simulink model "EvPowertrainController4EM"  (R2023a)
settings: configuration reference "VehicleFixed10ms" (kept outside this file)
model workspace (MAT data in the model file):
  CtrlVcuCnstrntPnltyFctr = 10000000
  CtrlVcuEMTrqSplitGrid = 200
  CtrlVcuPwrDeltaPnlty = 2
  CtrlVcuTracPwrErrPnlty = 6
  CtrlVcuTrqVecBrkThresh = 0.01
  CtrlVcuTrqVecIGain = 0
  CtrlVcuTrqVecMinTrq = 50
  CtrlVcuTrqVecPGain = -2000
  CtrlVcuTrqVecSteerThresh = 0.349065850399
  CtrlVcuTrqVecVelThresh = 2.5
undefined symbols (not defined in the file): CtrlVcuEvChrgLmtBpt, CtrlVcuEvRegenBrkCutOff, CtrlVcuEvRegenBrkSpdBpt, CtrlVcuEvSocBpt, eff, PlntBrkActrBoreFrnt, PlntBrkFrntBias, PlntBrkKinFricCffFrnt, PlntBrkNumPadsFrnt, PlntBrkPadMeanRadiusFrnt, PlntBrkPrsFctr, PlntBrkRearBias, PlntDiffrntl2Eff, PlntDiffrntl2Ratio, PlntDiffrntlEff, PlntDiffrntlRatio, PlntEM1EffTbl, PlntEM1Spd, PlntEM1Trq, PlntEM1TrqEff, PlntEM2EffTbl, PlntEM2Spd, PlntEM2Trq, PlntEM2TrqEff, PlntEM3EffTbl, PlntEM3Spd, PlntEM3Trq, PlntEM3TrqEff, PlntEMWhlGearEffFL, PlntEMWhlGearEffRL, PlntEMWhlGearRatioFL, PlntEMWhlGearRatioRL, PlntTransEffSpdBpt, PlntTransEffTbl, PlntTransEffTempBpt, PlntTransEffTrqBpt, PlntTransGearNumVect, PlntTransGearRatioVect, PlntVehDstCGFrntAxl, PlntVehDstCGRearAxl, PlntWhlLdRadius
libraries: simulink x13, autolibutils x2, slpidlib x2
(part 1 of 5)
settings Model: DataDictionary=VirtualVehicleTemplate.sldd  ModifiedByFormat=The MathWorks, Inc.  Creator=The MathWorks, Inc.  LastModifiedBy=The MathWorks, Inc.
settings ConfigSetRef: SourceName=VehicleFixed10ms

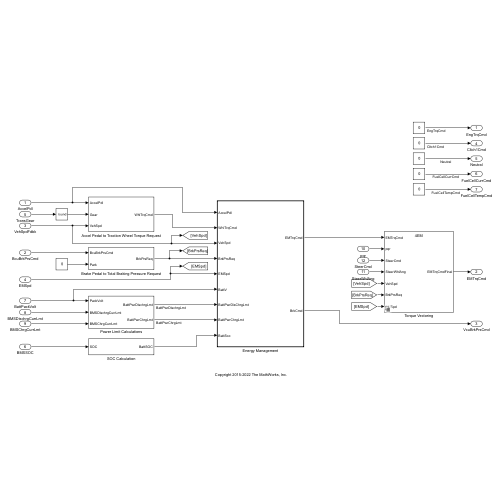
[thumbnail: Simulink's stored preview of the top-level diagram]
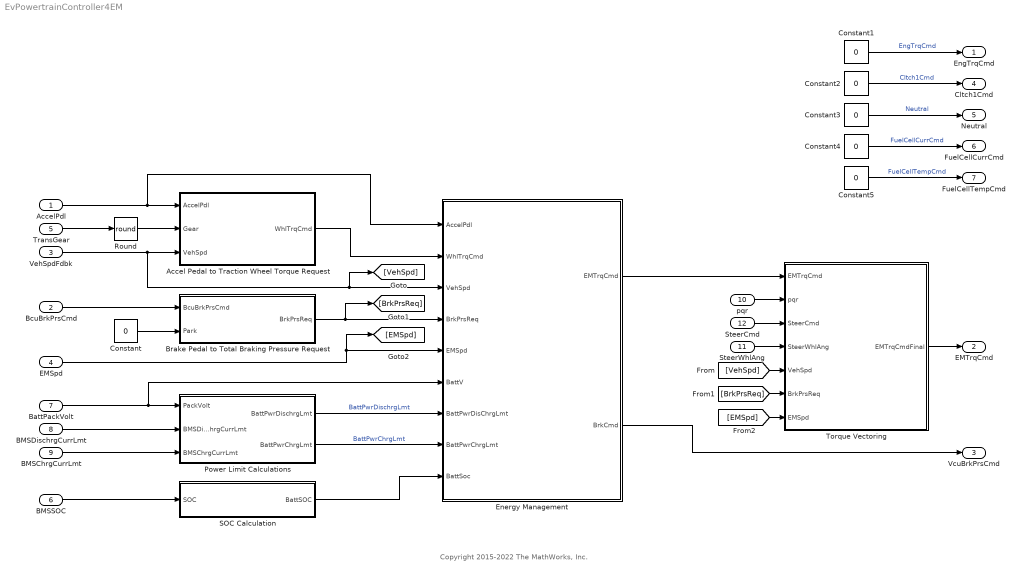
== system EvPowertrainController4EM ==
  note: Copyright 2015-2022 The MathWorks, Inc.
  AccelPdl : Inport  OutDataTypeStr=double  PortDimensions=1
  BcuBrkPrsCmd : Inport  Port=2  OutDataTypeStr=double  PortDimensions=4
  VehSpdFdbk : Inport  Port=3  OutDataTypeStr=double  PortDimensions=1
  EMSpd : Inport  Port=4  OutDataTypeStr=double
  TransGear : Inport  Port=5  OutDataTypeStr=double  PortDimensions=1
  BMSSOC : Inport  Port=6
  BattPackVolt : Inport  Port=7
  BMSDischrgCurrLmt : Inport  Port=8
  BMSChrgCurrLmt : Inport  Port=9
  pqr : Inport  Port=10  PortDimensions=3
  SteerWhlAng : Inport  Port=11  PortDimensions=4
  SteerCmd : Inport  Port=12
  Accel Pedal to Traction Wheel Torque Request : Subsystem  InitFcn=[~]=autosharedicon('autolibinternalvvblock',gcb,0);  VariantControl=Choice
  Brake Pedal to Total Braking Pressure Request : Subsystem  InitFcn=[~]=autosharedicon('autolibinternalvvblock',gcb,0);
  Constant : Constant  Value=0
  Constant{1..5} (5 alike) : Constant  Value=0  SampleTime=-1
  Energy Management : Subsystem  LoadFcn=[~]=autosharedicon('autolibinternalvvblock',gcb,0);  TreatAsAtomicUnit=on
  Power Limit Calculations : Subsystem  InitFcn=[~]=autosharedicon('autolibinternalvvblock',gcb,0);
  Round : Rounding  Operator=round
  SOC Calculation : Subsystem  InitFcn=[~]=autosharedicon('autolibinternalvvblock',gcb,0);
  Torque Vectoring : Subsystem  Variant=on  VariantControlMode=label  VariantControl=Choice  LabelModeActiveChoice=4EM
  EngTrqCmd : Outport  OutDataTypeStr=double  PortDimensions=1  VectorParamsAs1DForOutWhenUnconnected=off
  EMTrqCmd : Outport  Port=2  OutDataTypeStr=double  VectorParamsAs1DForOutWhenUnconnected=off
  VcuBrkPrsCmd : Outport  Port=3  OutDataTypeStr=double  PortDimensions=4  VectorParamsAs1DForOutWhenUnconnected=off
  Cltch1Cmd : Outport  Port=4  OutDataTypeStr=double  PortDimensions=1  VectorParamsAs1DForOutWhenUnconnected=off
  Neutral : Outport  Port=5  OutDataTypeStr=double  PortDimensions=1  VectorParamsAs1DForOutWhenUnconnected=off
  FuelCellCurrCmd : Outport  Port=6  OutDataTypeStr=double  PortDimensions=1
  FuelCellTempCmd : Outport  Port=7  OutDataTypeStr=double  PortDimensions=1
  wires:
  AccelPdl/1 -> Energy Management/1(AccelPdl), Accel Pedal to Traction Wheel Torque Request/1(AccelPdl)
  BcuBrkPrsCmd/1 -> Brake Pedal to Total Braking Pressure Request/1(BcuBrkPrsCmd)
  Energy Management/2(BrkCmd) -> VcuBrkPrsCmd/1
  Constant/1 -> Brake Pedal to Total Braking Pressure Request/2(Park)
  Brake Pedal to Total Braking Pressure Request/1(BrkPrsReq) -> [BrkPrsReq], Energy Management/4("BrkPrsReq ")
  VehSpdFdbk/1 -> [VehSpd], Energy Management/3(VehSpd), Accel Pedal to Traction Wheel Torque Request/3(VehSpd)
  Constant2/1 -> Cltch1Cmd/1  "Cltch1Cmd"
  Constant3/1 -> Neutral/1  "Neutral"
  Constant1/1 -> EngTrqCmd/1  "EngTrqCmd"
  Constant4/1 -> FuelCellCurrCmd/1  "FuelCellCurrCmd"
  Constant5/1 -> FuelCellTempCmd/1  "FuelCellTempCmd"
  Accel Pedal to Traction Wheel Torque Request/1(WhlTrqCmd) -> Energy Management/2(WhlTrqCmd)
  TransGear/1 -> Round/1
  Round/1 -> Accel Pedal to Traction Wheel Torque Request/2(Gear)
  BMSChrgCurrLmt/1 -> Power Limit Calculations/3(BMSChrgCurrLmt)
  BMSSOC/1 -> SOC Calculation/1(SOC)
  BattPackVolt/1 -> Energy Management/6(BattV), Power Limit Calculations/1(PackVolt)
  BMSDischrgCurrLmt/1 -> Power Limit Calculations/2(BMSDischrgCurrLmt)
  Power Limit Calculations/1(BattPwrDischrgLmt) -> Energy Management/7(BattPwrDisChrgLmt)  "BattPwrDischrgLmt"
  Power Limit Calculations/2(BattPwrChrgLmt) -> Energy Management/8("BattPwrChrgLmt ")  "BattPwrChrgLmt"
  SOC Calculation/1(BattSOC) -> Energy Management/9(BattSoc)
  EMSpd/1 -> [EMSpd], Energy Management/5(EMSpd)
  Energy Management/1(EMTrqCmd) -> Torque Vectoring/1(EMTrqCmd)
  pqr/1 -> Torque Vectoring/2(pqr)
  SteerCmd/1 -> Torque Vectoring/3(SteerCmd)
  SteerWhlAng/1 -> Torque Vectoring/4(SteerWhlAng)
  [VehSpd] -> Torque Vectoring/5(VehSpd)
  [BrkPrsReq] -> Torque Vectoring/6(BrkPrsReq)
  [EMSpd] -> Torque Vectoring/7(EMSpd)
  Torque Vectoring/1(EMTrqCmdFinal) -> EMTrqCmd/1

== system EvPowertrainController4EM/Accel Pedal to Traction Wheel Torque Request ==
  note: Convert Accelerator Pedal Position to
      | Wheel Torque Command using Motor
      | Torque Speed Curves.
      |
      | Can be replaced with 2D Lookup Table
      | with AccelPdl and VehSpd as inputs and
      | Motor or Wheel Torque Command as output.
  AccelPdl : Inport
  Gear : Inport  Port=2
  VehSpd : Inport  Port=3
  EM2WhlTrq : Subsystem  Variant=on  VariantControlMode=label  VariantControl=Choice  LabelModeActiveChoice=4EM
  Product1 : Product
  WhlTrqCmd : Outport  VectorParamsAs1DForOutWhenUnconnected=off
  wires:
  Product1/1 -> WhlTrqCmd/1
  AccelPdl/1 -> Product1/1
  Gear/1 -> EM2WhlTrq/1(Gear)
  VehSpd/1 -> EM2WhlTrq/2(VehSpd)
  EM2WhlTrq/1(WhlTrqCmd) -> Product1/2

== system EvPowertrainController4EM/Brake Pedal to Total Braking Pressure Request ==
  BcuBrkPrsCmd : Inport
  Park : Inport  Port=2
  Front Bias : Constant  Value=PlntBrkFrntBias
  Gain4 : Gain  Gain=PlntBrkPrsFctr
  Mux : Mux
  Product : Product
  Rear Bias : Constant  Value=PlntBrkRearBias
  Terminator : Terminator
  BrkPrsReq : Outport  VectorParamsAs1DForOutWhenUnconnected=off
  wires:
  BcuBrkPrsCmd/1 -> Product/2
  Mux/1 -> Product/1
  Rear Bias/1 -> Mux/4, Mux/3
  Front Bias/1 -> Mux/1, Mux/2
  Gain4/1 -> BrkPrsReq/1
  Product/1 -> Gain4/1
  Park/1 -> Terminator/1

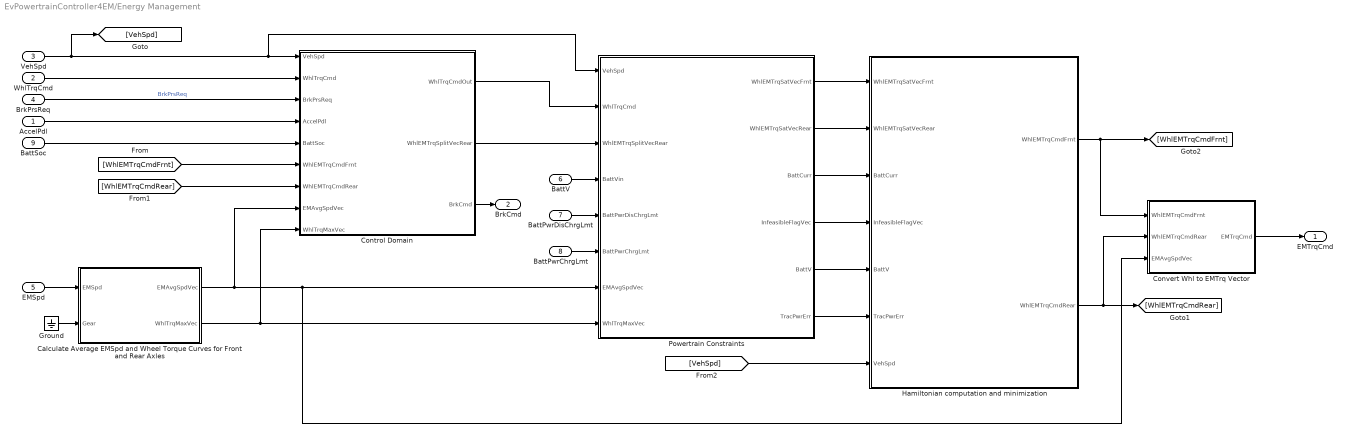
== system EvPowertrainController4EM/Energy Management ==
  AccelPdl : Inport
  WhlTrqCmd : Inport  Port=2
  VehSpd : Inport  Port=3
  "BrkPrsReq " : Inport  Port=4
  EMSpd : Inport  Port=5
  BattV : Inport  Port=6
  BattPwrDisChrgLmt : Inport  Port=7
  "BattPwrChrgLmt " : Inport  Port=8
  BattSoc : Inport  Port=9
  Calculate Average EMSpd and Wheel Torque Curves for Front and Rear Axles : Subsystem  Variant=on  VariantControlMode=label  VariantControl=Choice  LabelModeActiveChoice=4EM
  "Control Domain " : Subsystem  InitFcn="[~] =  autosharedeval('1');"
  Convert Whl to EMTrq Vector : Subsystem  Variant=on  VariantControlMode=label  VariantControl=Choice  LabelModeActiveChoice=4EM
  Ground : Ground
  Hamiltonian computation and minimization : Subsystem  InitFcn="[~] =  autosharedeval('1');"
  "Powertrain Constraints " : Subsystem  InitFcn="[~] =  autosharedeval('1');"
  EMTrqCmd : Outport  VectorParamsAs1DForOutWhenUnconnected=off
  BrkCmd : Outport  Port=2  VectorParamsAs1DForOutWhenUnconnected=off
  wires:
  "Control Domain "/1(WhlTrqCmdOut) -> "Powertrain Constraints "/2(WhlTrqCmd)
  "BrkPrsReq "/1 -> "Control Domain "/3("BrkPrsReq ")  "BrkPrsReq"
  AccelPdl/1 -> "Control Domain "/4(AccelPdl)
  "Control Domain "/3(BrkCmd) -> BrkCmd/1
  "Powertrain Constraints "/6(TracPwrErr) -> Hamiltonian computation and minimization/6(TracPwrErr)
  BattV/1 -> "Powertrain Constraints "/4(BattVin)
  VehSpd/1 -> [VehSpd], "Control Domain "/1(VehSpd), "Powertrain Constraints "/1(VehSpd)
  Hamiltonian computation and minimization/2(WhlEMTrqCmdRear) -> [WhlEMTrqCmdRear], Convert Whl to EMTrq Vector/2(WhlEMTrqCmdRear)
  Hamiltonian computation and minimization/1(WhlEMTrqCmdFrnt) -> [WhlEMTrqCmdFrnt], Convert Whl to EMTrq Vector/1(WhlEMTrqCmdFrnt)
  "Powertrain Constraints "/4(InfeasibleFlagVec) -> Hamiltonian computation and minimization/4(InfeasibleFlagVec)
  "Powertrain Constraints "/3(BattCurr) -> Hamiltonian computation and minimization/3(BattCurr)
  "Powertrain Constraints "/5(BattV) -> Hamiltonian computation and minimization/5(BattV)
  WhlTrqCmd/1 -> "Control Domain "/2(WhlTrqCmd)
  "Control Domain "/2(WhlEMTrqSplitVecRear) -> "Powertrain Constraints "/3(WhlEMTrqSplitVecRear)
  Calculate Average EMSpd and Wheel Torque Curves for Front and Rear Axles/1(EMAvgSpdVec) -> Convert Whl to EMTrq Vector/3(EMAvgSpdVec), "Powertrain Constraints "/7(EMAvgSpdVec), "Control Domain "/8(EMAvgSpdVec)
  "BattPwrChrgLmt "/1 -> "Powertrain Constraints "/6("BattPwrChrgLmt ")
  BattPwrDisChrgLmt/1 -> "Powertrain Constraints "/5(BattPwrDisChrgLmt)
  [WhlEMTrqCmdFrnt] -> "Control Domain "/6(WhlEMTrqCmdFrnt)
  BattSoc/1 -> "Control Domain "/5(BattSoc)
  EMSpd/1 -> Calculate Average EMSpd and Wheel Torque Curves for Front and Rear Axles/1(EMSpd)
  Convert Whl to EMTrq Vector/1(EMTrqCmd) -> EMTrqCmd/1
  [WhlEMTrqCmdRear] -> "Control Domain "/7(WhlEMTrqCmdRear)
  Ground/1 -> Calculate Average EMSpd and Wheel Torque Curves for Front and Rear Axles/2(Gear)
  Calculate Average EMSpd and Wheel Torque Curves for Front and Rear Axles/2(WhlTrqMaxVec) -> "Powertrain Constraints "/8(WhlTrqMaxVec), "Control Domain "/9(WhlTrqMaxVec)
  "Powertrain Constraints "/1(WhlEMTrqSatVecFrnt) -> Hamiltonian computation and minimization/1(WhlEMTrqSatVecFrnt)
  "Powertrain Constraints "/2(WhlEMTrqSatVecRear) -> Hamiltonian computation and minimization/2(WhlEMTrqSatVecRear)
  [VehSpd] -> Hamiltonian computation and minimization/7(VehSpd)

== system EvPowertrainController4EM/Power Limit Calculations ==
  note: BMS has opposite sign convention for current
  note: Use Current Limits from BMS to calculate
      | discharge and charge power limits
  PackVolt : Inport
  BMSDischrgCurrLmt : Inport  Port=2
  BMSChrgCurrLmt : Inport  Port=3
  Data Type Conversion : DataTypeConversion  SaturateOnIntegerOverflow=off  RndMeth=Floor
  Data Type Conversion1 : DataTypeConversion  SaturateOnIntegerOverflow=off  RndMeth=Floor
  Gain : Gain  Gain=-1
  Gain1 : Gain  Gain=-1
  Product : Product
  Product1 : Product
  BattPwrDischrgLmt : Outport  VectorParamsAs1DForOutWhenUnconnected=off
  BattPwrChrgLmt : Outport  Port=2  VectorParamsAs1DForOutWhenUnconnected=off
  wires:
  Gain/1 -> Product1/2
  Gain1/1 -> Product/2
  Product/1 -> Data Type Conversion1/1
  Product1/1 -> Data Type Conversion/1
  PackVolt/1 -> Product/1, Product1/1
  BMSChrgCurrLmt/1 -> Gain/1
  BMSDischrgCurrLmt/1 -> Gain1/1
  Data Type Conversion/1 -> BattPwrChrgLmt/1
  Data Type Conversion1/1 -> BattPwrDischrgLmt/1

== system EvPowertrainController4EM/SOC Calculation ==
  SOC : Inport
  Data Type Conversion : DataTypeConversion  SaturateOnIntegerOverflow=off  RndMeth=Floor
  convert2percent : Gain  Gain=100
  BattSOC : Outport
  wires:
  convert2percent/1 -> Data Type Conversion/1
  SOC/1 -> convert2percent/1
  Data Type Conversion/1 -> BattSOC/1

== system EvPowertrainController4EM/Torque Vectoring ==
  EMTrqCmd : Inport
  pqr : Inport  Port=2
  SteerCmd : Inport  Port=3
  SteerWhlAng : Inport  Port=4
  VehSpd : Inport  Port=5
  BrkPrsReq : Inport  Port=6
  EMSpd : Inport  Port=7
  3EM : Subsystem  LoadFcn=[~]=autosharedicon('autolibinternalvvblock',gcb,0);  VariantControl=3EM
  4EM : Subsystem  LoadFcn=[~]=autosharedicon('autolibinternalvvblock',gcb,0);  VariantControl=4EM
  No Torque Vectoring : Subsystem  VariantControl=No Torque Vectoring
  EMTrqCmdFinal : Outport

== system EvPowertrainController4EM/Accel Pedal to Traction Wheel Torque Request/EM2WhlTrq ==
  Gear : Inport
  VehSpd : Inport  Port=2
  2EM : Subsystem  VariantControl=2EM
  3EM Dual Front : Subsystem  VariantControl=3EM Dual Front
  3EM Dual Rear : Subsystem  VariantControl=3EM Dual Rear
  4EM : Subsystem  VariantControl=4EM
  WhlTrqCmd : Outport

== system EvPowertrainController4EM/Energy Management/Calculate Average EMSpd and Wheel Torque Curves for Front and Rear Axles ==
  EMSpd : Inport
  Gear : Inport  Port=2
  2EM : Subsystem  VariantControl=2EM
  3EM Dual Front : Subsystem  VariantControl=3EM Dual Front
  3EM Dual Rear : Subsystem  VariantControl=3EM Dual Rear
  4EM : Subsystem  VariantControl=4EM
  EMAvgSpdVec : Outport
  WhlTrqMaxVec : Outport  Port=2

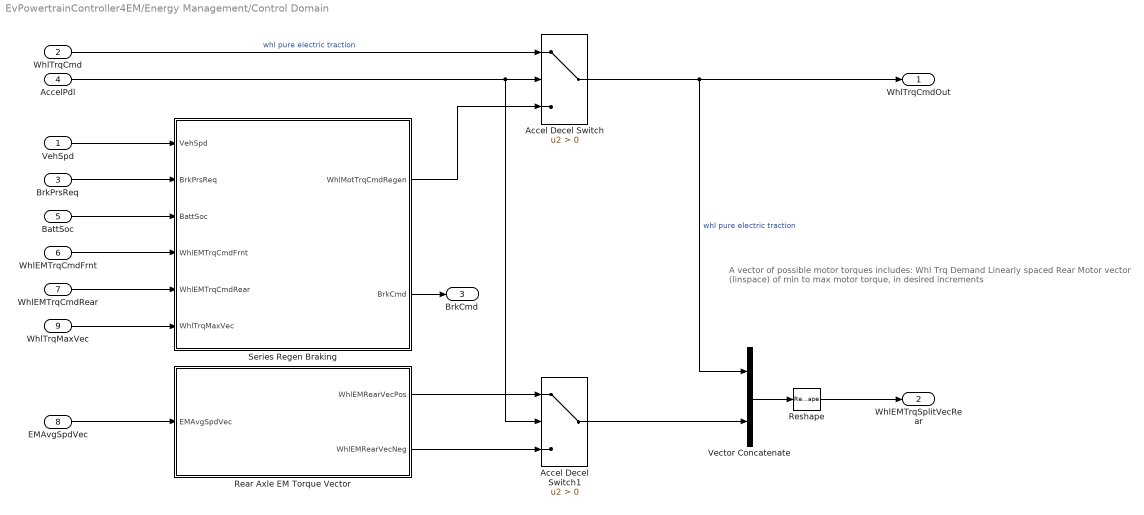
== system EvPowertrainController4EM/Energy Management/Control Domain  ==
  note: A vector of possible motor torques includes:
      | Whl Trq Demand
      | Linearly spaced Rear Motor vector (linspace) of min to max motor torque, in desired increments
  VehSpd : Inport
  WhlTrqCmd : Inport  Port=2
  "BrkPrsReq " : Inport  Port=3
  AccelPdl : Inport  Port=4
  BattSoc : Inport  Port=5
  WhlEMTrqCmdFrnt : Inport  Port=6
  WhlEMTrqCmdRear : Inport  Port=7
  EMAvgSpdVec : Inport  Port=8
  WhlTrqMaxVec : Inport  Port=9
  Accel Decel Switch : Switch  Criteria=u2 > Threshold  SaturateOnIntegerOverflow=off  InputSameDT=off
  Accel Decel Switch1 : Switch  Criteria=u2 > Threshold  SaturateOnIntegerOverflow=off  InputSameDT=off
  Rear Axle EM Torque Vector : Subsystem  Variant=on  VariantControlMode=label  VariantControl=Choice  LabelModeActiveChoice=3EM Dual Rear or 4EM
  Reshape : Reshape
  Series Regen Braking : Subsystem  InitFcn=%[~]=autosharedicon('autolibutils',gcb,0);  VariantControl=Variant
  Vector Concatenate : Concatenate
  WhlTrqCmdOut : Outport  VectorParamsAs1DForOutWhenUnconnected=off
  WhlEMTrqSplitVecRear : Outport  Port=2  VectorParamsAs1DForOutWhenUnconnected=off
  BrkCmd : Outport  Port=3  VectorParamsAs1DForOutWhenUnconnected=off
  wires:
  Vector Concatenate/1 -> Reshape/1
  Reshape/1 -> WhlEMTrqSplitVecRear/1
  WhlTrqMaxVec/1 -> Series Regen Braking/6(WhlTrqMaxVec)
  AccelPdl/1 -> Accel Decel Switch1/2, Accel Decel Switch/2
  Series Regen Braking/2(" BrkCmd") -> BrkCmd/1
  WhlTrqCmd/1 -> Accel Decel Switch/1  "whl pure electric traction"
  "BrkPrsReq "/1 -> Series Regen Braking/2("BrkPrsReq ")
  EMAvgSpdVec/1 -> Rear Axle EM Torque Vector/1(EMAvgSpdVec)
  VehSpd/1 -> Series Regen Braking/1(VehSpd)
  Accel Decel Switch/1 -> Vector Concatenate/1, WhlTrqCmdOut/1  "whl pure electric traction"
  Accel Decel Switch1/1 -> Vector Concatenate/2
  Series Regen Braking/1(" WhlMotTrqCmdRegen") -> Accel Decel Switch/3
  WhlEMTrqCmdFrnt/1 -> Series Regen Braking/4(WhlEMTrqCmdFrnt)
  WhlEMTrqCmdRear/1 -> Series Regen Braking/5(WhlEMTrqCmdRear)
  BattSoc/1 -> Series Regen Braking/3(BattSoc)
  Rear Axle EM Torque Vector/1(WhlEMRearVecPos) -> Accel Decel Switch1/1
  Rear Axle EM Torque Vector/2(WhlEMRearVecNeg) -> Accel Decel Switch1/3

== system EvPowertrainController4EM/Energy Management/Convert Whl to EMTrq Vector ==
  WhlEMTrqCmdFrnt : Inport
  WhlEMTrqCmdRear : Inport  Port=2
  EMAvgSpdVec : Inport  Port=3
  2EM : Subsystem  VariantControl=2EM
  3EM Dual Front : Subsystem  VariantControl=3EM Dual Front
  3EM Dual Rear : Subsystem  VariantControl=3EM Dual Rear
  4EM : Subsystem  VariantControl=4EM
  EMTrqCmd : Outport

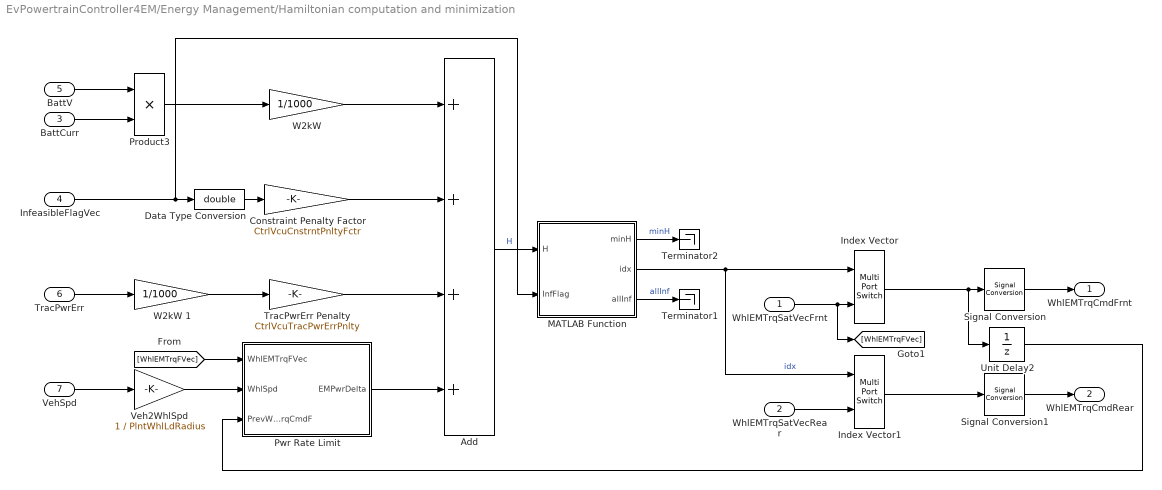
== system EvPowertrainController4EM/Energy Management/Hamiltonian computation and minimization ==
  WhlEMTrqSatVecFrnt : Inport
  WhlEMTrqSatVecRear : Inport  Port=2
  BattCurr : Inport  Port=3
  InfeasibleFlagVec : Inport  Port=4
  BattV : Inport  Port=5
  TracPwrErr : Inport  Port=6
  VehSpd : Inport  Port=7
  Add : Sum  Inputs=++++
  Constraint Penalty Factor : Gain  Gain=CtrlVcuCnstrntPnltyFctr
  Data Type Conversion : DataTypeConversion  OutDataTypeStr=double  SaturateOnIntegerOverflow=off  RndMeth=Floor
  Index Vector : MultiPortSwitch  Inputs=1  SaturateOnIntegerOverflow=off  InputSameDT=off
  Index Vector1 : MultiPortSwitch  Inputs=1  SaturateOnIntegerOverflow=off  InputSameDT=off
  MATLAB Function : MATLAB Function  InitFcn="[~] =  autosharedeval('1');"  TreatAsAtomicUnit=on
  Product3 : Product
  Pwr Rate Limit : Subsystem  InitFcn="[~] =  autosharedeval('1');"
  Signal Conversion : SignalConversion  OverrideOpt=off
  Signal Conversion1 : SignalConversion  OverrideOpt=off
  Terminator1 : Terminator
  Terminator2 : Terminator
  TracPwrErr Penalty : Gain  Gain=CtrlVcuTracPwrErrPnlty
  Unit Delay2 : UnitDelay  SampleTime=-1  HasFrameUpgradeWarning=on
  Veh2WhlSpd : Gain  Gain=1 / PlntWhlLdRadius
  "W2kW " : Gain  Gain=1/1000
  W2kW 1 : Gain  Gain=1/1000
  WhlEMTrqCmdFrnt : Outport  VectorParamsAs1DForOutWhenUnconnected=off
  WhlEMTrqCmdRear : Outport  Port=2  VectorParamsAs1DForOutWhenUnconnected=off
  wires:
  Constraint Penalty Factor/1 -> Add/2
  TracPwrErr Penalty/1 -> Add/3
  W2kW 1/1 -> TracPwrErr Penalty/1
  TracPwrErr/1 -> W2kW 1/1
  Signal Conversion1/1 -> WhlEMTrqCmdRear/1
  Signal Conversion/1 -> WhlEMTrqCmdFrnt/1
  Index Vector/1 -> Unit Delay2/1, Signal Conversion/1
  "W2kW "/1 -> Add/1
  BattV/1 -> Product3/1
  BattCurr/1 -> Product3/2
  Index Vector1/1 -> Signal Conversion1/1
  Add/1 -> MATLAB Function/1(H)  "H"
  MATLAB Function/1(minH) -> Terminator2/1  "minH"
  MATLAB Function/2(idx) -> Index Vector1/1, Index Vector/1  "idx"
  WhlEMTrqSatVecRear/1 -> Index Vector1/2
  InfeasibleFlagVec/1 -> Data Type Conversion/1, MATLAB Function/2(InfFlag)
  WhlEMTrqSatVecFrnt/1 -> Index Vector/2, [WhlEMTrqFVec]
  Product3/1 -> "W2kW "/1
  [WhlEMTrqFVec] -> Pwr Rate Limit/1(WhlEMTrqFVec)
  Veh2WhlSpd/1 -> Pwr Rate Limit/2(WhlSpd)
  Unit Delay2/1 -> Pwr Rate Limit/3(PrevWhlEMTrqCmdF)
  MATLAB Function/3(allInf) -> Terminator1/1  "allInf"
  Pwr Rate Limit/1(EMPwrDelta) -> Add/4
  Data Type Conversion/1 -> Constraint Penalty Factor/1
  VehSpd/1 -> Veh2WhlSpd/1

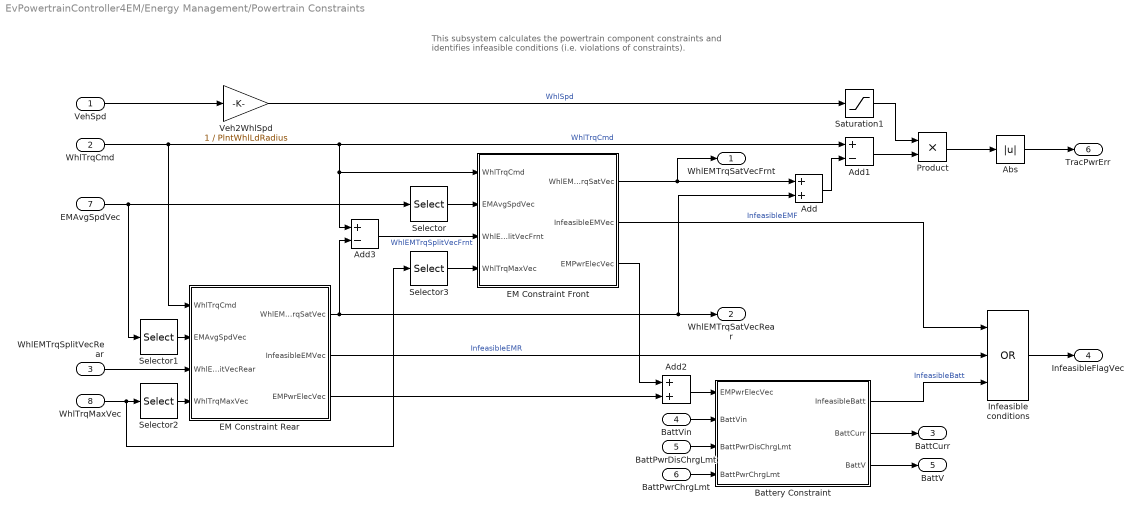
== system EvPowertrainController4EM/Energy Management/Powertrain Constraints  ==
  note: This subsystem calculates the powertrain component constraints
      | and identifies infeasible conditions (i.e. violations of constraints).
  VehSpd : Inport
  WhlTrqCmd : Inport  Port=2
  WhlEMTrqSplitVecRear : Inport  Port=3
  BattVin : Inport  Port=4
  BattPwrDisChrgLmt : Inport  Port=5
  "BattPwrChrgLmt " : Inport  Port=6
  EMAvgSpdVec : Inport  Port=7
  WhlTrqMaxVec : Inport  Port=8
  Abs : Abs  SaturateOnIntegerOverflow=off
  Add : Sum
  Add1 : Sum  Inputs=+-
  Add2 : Sum
  Add3 : Sum  Inputs=+-
  Battery Constraint : Subsystem  InitFcn="[~] =  autosharedeval('1');"
  EM Constraint Front : Subsystem  InitFcn="[~] =  autosharedeval('1');"
  EM Constraint Rear : Subsystem  InitFcn="[~] =  autosharedeval('1');"
  Infeasible conditions : Logic  Operator=OR  Inputs=3  AllPortsSameDT=off  OutDataTypeStr=boolean
  Product : Product
  Saturation1 : Saturate  UpperLimit=inf  LowerLimit=0.001
  Selector : Selector  InputPortWidth=2  IndexOptions=Index vector (dialog)  Indices=[1]  OutputSizes=1
  Selector1 : Selector  InputPortWidth=2  IndexOptions=Index vector (dialog)  Indices=[2]  OutputSizes=1
  Selector2 : Selector  InputPortWidth=2  IndexOptions=Index vector (dialog)  Indices=[2]  OutputSizes=1
  Selector3 : Selector  InputPortWidth=2  IndexOptions=Index vector (dialog)  Indices=[1]  OutputSizes=1
  Veh2WhlSpd : Gain  Gain=1 / PlntWhlLdRadius
  WhlEMTrqSatVecFrnt : Outport  VectorParamsAs1DForOutWhenUnconnected=off
  WhlEMTrqSatVecRear : Outport  Port=2  VectorParamsAs1DForOutWhenUnconnected=off
  BattCurr : Outport  Port=3  VectorParamsAs1DForOutWhenUnconnected=off
  InfeasibleFlagVec : Outport  Port=4  VectorParamsAs1DForOutWhenUnconnected=off
  BattV : Outport  Port=5  VectorParamsAs1DForOutWhenUnconnected=off
  TracPwrErr : Outport  Port=6  VectorParamsAs1DForOutWhenUnconnected=off
  wires:
  EM Constraint Rear/1(WhlEMTrqSatVec) -> WhlEMTrqSatVecRear/1, Add/2, Add3/2
  Add/1 -> Add1/2
  Add1/1 -> Product/2
  Battery Constraint/1(InfeasibleBatt) -> Infeasible conditions/3  "InfeasibleBatt"
  Infeasible conditions/1 -> InfeasibleFlagVec/1
  EM Constraint Rear/2(InfeasibleEMVec) -> Infeasible conditions/2  "InfeasibleEMR"
  Abs/1 -> TracPwrErr/1
  Veh2WhlSpd/1 -> Saturation1/1  "WhlSpd"
  Saturation1/1 -> Product/1
  BattVin/1 -> Battery Constraint/2(BattVin)
  WhlTrqCmd/1 -> EM Constraint Rear/1(WhlTrqCmd), Add1/1, EM Constraint Front/1(WhlTrqCmd), Add3/1  "WhlTrqCmd"
  WhlEMTrqSplitVecRear/1 -> EM Constraint Rear/3(WhlEMTrqSplitVecRear)
  EM Constraint Front/1(WhlEMTrqSatVec) -> WhlEMTrqSatVecFrnt/1, Add/1
  Battery Constraint/2(BattCurr) -> BattCurr/1
  EM Constraint Front/2(InfeasibleEMVec) -> Infeasible conditions/1  "InfeasibleEMF"
  Add2/1 -> Battery Constraint/1(EMPwrElecVec)
  VehSpd/1 -> Veh2WhlSpd/1
  EM Constraint Rear/3(EMPwrElecVec) -> Add2/2
  Battery Constraint/3(BattV) -> BattV/1
  EMAvgSpdVec/1 -> Selector/1, Selector1/1
  Add3/1 -> EM Constraint Front/3(WhlEMTrqSplitVecFrnt)  "WhlEMTrqSplitVecFrnt"
  Product/1 -> Abs/1
  EM Constraint Front/3(EMPwrElecVec) -> Add2/1
  "BattPwrChrgLmt "/1 -> Battery Constraint/4("BattPwrChrgLmt ")
  BattPwrDisChrgLmt/1 -> Battery Constraint/3(BattPwrDisChrgLmt)
  WhlTrqMaxVec/1 -> Selector3/1, Selector2/1
  Selector/1 -> EM Constraint Front/2(EMAvgSpdVec)
  Selector1/1 -> EM Constraint Rear/2(EMAvgSpdVec)
  Selector2/1 -> EM Constraint Rear/4(WhlTrqMaxVec)
  Selector3/1 -> EM Constraint Front/4(WhlTrqMaxVec)

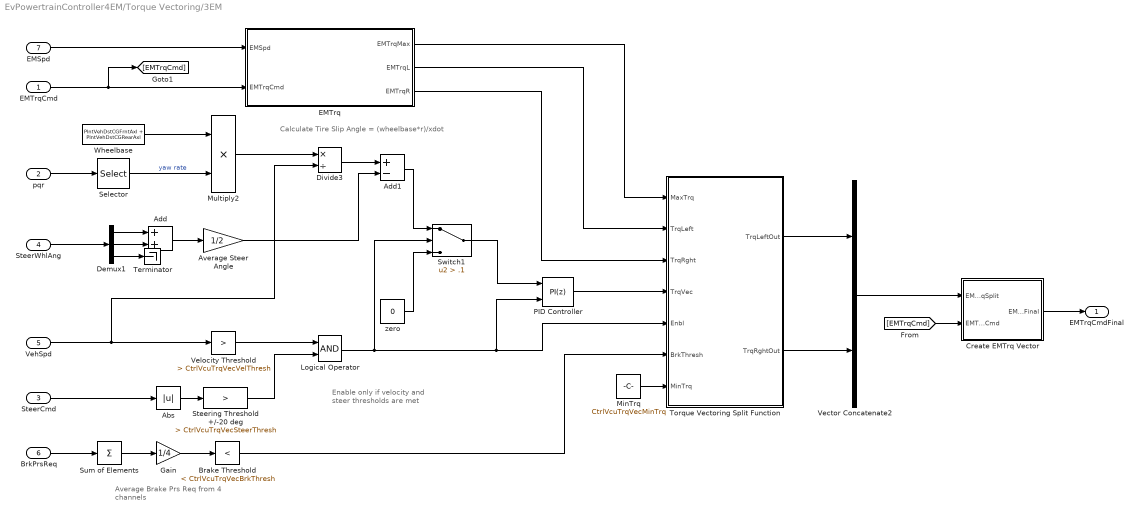
== system EvPowertrainController4EM/Torque Vectoring/3EM ==
  note: Calculate Tire Slip Angle = (wheelbase*r)/xdot
  note: Enable only if velocity and
      | steer thresholds are met
  note: Average Brake Prs Req
      | from 4 channels
  EMTrqCmd : Inport
  pqr : Inport  Port=2
  SteerCmd : Inport  Port=3
  SteerWhlAng : Inport  Port=4
  VehSpd : Inport  Port=5
  BrkPrsReq : Inport  Port=6
  EMSpd : Inport  Port=7
  Abs : Abs  SaturateOnIntegerOverflow=off
  Add : Sum
  Add1 : Sum  Inputs=+-
  Average Steer Angle : Gain  Gain=1/2
  Brake Threshold : simulink/Logic and Bit Operations/Compare To Constant  relop=<  const=CtrlVcuTrqVecBrkThresh  OutDataTypeStr=boolean
  Create EMTrq Vector : Subsystem  Variant=on  VariantControlMode=label  VariantControl=Choice  LabelModeActiveChoice=3EMDualRear
  Demux1 : Demux  Outputs=[1 1 2]
  Divide3 : Product  Inputs=*/
  EMTrq : Subsystem  Variant=on  VariantControlMode=label  VariantControl=Choice  LabelModeActiveChoice=3EMDualRear
  Gain : Gain  Gain=1/4
  Logical Operator : Logic  AllPortsSameDT=off  OutDataTypeStr=boolean
  MinTrq : Constant  Value=CtrlVcuTrqVecMinTrq  SampleTime=-1
  Multiply2 : Product
  PID Controller : slpidlib/PID Controller  Controller=PI  Form=Parallel  TimeDomain=Discrete-time  UseExternalTs=off  SampleTime=-1  IntegratorMethod=Forward Euler  FilterMethod=Forward Euler  ControllerParametersSource=internal  P=CtrlVcuTrqVecPGain  I=CtrlVcuTrqVecPGain  UseKiTs=off  D=0  N=1  UseFilter=on  TunerSelectOption=Transfer Function Based (PID Tuner App)  ZeroCross=off  InitialConditionSource=internal  InitialConditionForIntegrator=0  InitialConditionForFilter=0  DifferentiatorICPrevScaledInput=0  ExternalReset=either  TrackingMode=off  Kt=1  LimitOutput=off  SatLimitsSource=internal  UpperSaturationLimit=inf  LowerSaturationLimit=-inf  LinearizeAsGain=on  AntiWindupMode=none  Kb=1  LimitIntegrator=off  UpperIntegratorSaturationLimit=inf  LowerIntegratorSaturationLimit=-inf  POutMin=[]  POutMax=[]  IOutMin=[]  IOutMax=[]  DOutMin=[]  DOutMax=[]  NOutMin=[]  NOutMax=[]  SumOutMin=[]  SumOutMax=[]  SaturationOutMin=[]  SaturationOutMax=[]  PParamMin=[]  PParamMax=[]  IParamMin=[]  IParamMax=[]  DParamMin=[]  DParamMax=[]  NParamMin=[]  NParamMax=[]  KbParamMin=[]  KbParamMax=[]  KtParamMin=[]  KtParamMax=[]  KbOutMin=[]  KbOutMax=[]  KtOutMin=[]  KtOutMax=[]  IntegratorOutMin=[]  IntegratorOutMax=[]  FilterOutMin=[]  FilterOutMax=[]  SumI1OutMin=[]  SumI1OutMax=[]  SumI2OutMin=[]  SumI2OutMax=[]  SumI3OutMin=[]  SumI3OutMax=[]  SumI4OutMin=[]  SumI4OutMax=[]  SumDOutMin=[]  SumDOutMax=[]  DifferentiatorOutMin=[]  DifferentiatorOutMax=[]  FilterDiffOutCoefMin=[]  FilterDiffOutCoefMax=[]  ReciprocalOutMin=[]  ReciprocalOutMax=[]  SumDenOutMin=[]  SumDenOutMax=[]  SumNumOutMin=[]  SumNumOutMax=[]  DivideOutMin=[]  DivideOutMax=[]  UdiffTsProdOutMin=[]  UdiffTsProdOutMax=[]  NTsProdOutMin=[]  NTsProdOutMax=[]  UintegralTsProdOutMin=[]  UintegralTsProdOutMax=[]  UngainTsProdOutMin=[]  UngainTsProdOutMax=[]  ClampingZeroOutDataTypeStr=Inherit: Inherit via back propagation  ClampingZeroOutMin=[]  ClampingZeroOutMax=[]  FilterDenConstantOutDataTypeStr=Inherit: Inherit via back propagation  FilterDenConstantOutMin=[]  FilterDenConstantOutMax=[]  PCopyOutDataTypeStr=Inherit: Inherit via back propagation  PCopyOutMin=[]  PCopyOutMax=[]  NCopyOutDataTypeStr=Inherit: Inherit via back propagation  NCopyOutMin=[]  NCopyOutMax=[]  IntegratorContinuousStateAttributes=''  IntegratorStateMustResolveToSignalObject=off  IntegratorRTWStateStorageClass=Auto  FilterContinuousStateAttributes=''  FilterStateMustResolveToSignalObject=off  FilterRTWStateStorageClass=Auto  ParallelPVariant=InternalParameters  IdealPVariant=Disabled  IVariant=InternalParameters  DVariant=Disabled  IntegratorVariant=Discrete  SatVariant=Disabled  AWVariant=Passthrough  PCopyVariant=Disabled  TRVariant=Disabled  FdbkBlocksVariant=Forward  IdealPFdbkVariant=Disabled  SatFdbkVariant=Disabled  DerivativeFilterVariant=Disabled  NVariant=Disabled  NCopyVariant=Disabled_SignalSpec  FilterICVariant=Disabled  IntegratorICVariant=InternalICs  ExternalResetVariant=ExternalReset  TRSumVariant=Passthrough  SumFdbkVariant=Disabled  SumVariant=Sum_PI  TsampFilterVariant=InternalTs  TsampNgainVariant=Passthrough  TsampIntegralVariant=Disabled_SignalSpec  ExternalSaturationOutDataTypeStr=Inherit: Same as second input
  Selector : Selector  InputPortWidth=3  IndexOptions=Index vector (dialog)  Indices=[3]  OutputSizes=1
  Steering Threshold +/-20 deg : simulink/Logic and Bit Operations/Compare To Constant  relop=>  const=CtrlVcuTrqVecSteerThresh  OutDataTypeStr=boolean
  Sum of Elements : Sum  Inputs=+
  Switch1 : Switch  Criteria=u2 > Threshold  Threshold=.1  SaturateOnIntegerOverflow=off  InputSameDT=off
  Terminator : Terminator
  Torque Vectoring Split Function : MATLAB Function  TreatAsAtomicUnit=on
  Vector Concatenate2 : Concatenate
  Velocity Threshold : simulink/Logic and Bit Operations/Compare To Constant  relop=>  const=CtrlVcuTrqVecVelThresh  OutDataTypeStr=boolean
  Wheelbase : Constant  Value=PlntVehDstCGFrntAxl + PlntVehDstCGRearAxl  SampleTime=-1
  zero : Constant  Value=0  SampleTime=-1
  EMTrqCmdFinal : Outport  VectorParamsAs1DForOutWhenUnconnected=off
  wires:
  Selector/1 -> Multiply2/2  "yaw rate"
  Gain/1 -> Brake Threshold/1
  Sum of Elements/1 -> Gain/1
  [EMTrqCmd] -> Create EMTrq Vector/2(EMTrqCmd)
  Vector Concatenate2/1 -> Create EMTrq Vector/1(EMTrqSplit)
  EMTrq/3(EMTrqR) -> Torque Vectoring Split Function/3(TrqRght)
  EMTrq/2(EMTrqL) -> Torque Vectoring Split Function/2(TrqLeft)
  EMTrq/1(EMTrqMax) -> Torque Vectoring Split Function/1(MaxTrq)
  EMSpd/1 -> EMTrq/1(EMSpd)
  Add1/1 -> Switch1/1
  SteerWhlAng/1 -> Demux1/1
  pqr/1 -> Selector/1
  zero/1 -> Switch1/3
  Demux1/1 -> Add/1
  Velocity Threshold/1 -> Logical Operator/1
  Abs/1 -> Steering Threshold +/-20 deg/1
  Torque Vectoring Split Function/1(TrqLeftOut) -> Vector Concatenate2/1
  Steering Threshold +/-20 deg/1 -> Logical Operator/2
  Add/1 -> Average Steer Angle/1
  Torque Vectoring Split Function/2(TrqRghtOut) -> Vector Concatenate2/2
  Logical Operator/1 -> Switch1/2, PID Controller/2, Torque Vectoring Split Function/5(Enbl)
  Brake Threshold/1 -> Torque Vectoring Split Function/6(BrkThresh)
  PID Controller/1 -> Torque Vectoring Split Function/4(TrqVec)
  Average Steer Angle/1 -> Add1/2
  Multiply2/1 -> Divide3/1
  VehSpd/1 -> Divide3/2, Velocity Threshold/1
  Demux1/2 -> Add/2
  SteerCmd/1 -> Abs/1
  Switch1/1 -> PID Controller/1
  Divide3/1 -> Add1/1
  BrkPrsReq/1 -> Sum of Elements/1
  Demux1/3 -> Terminator/1
  Wheelbase/1 -> Multiply2/1
  MinTrq/1 -> Torque Vectoring Split Function/7(MinTrq)
  Create EMTrq Vector/1(EMTrqCmdFinal) -> EMTrqCmdFinal/1
  EMTrqCmd/1 -> EMTrq/2(EMTrqCmd), [EMTrqCmd]

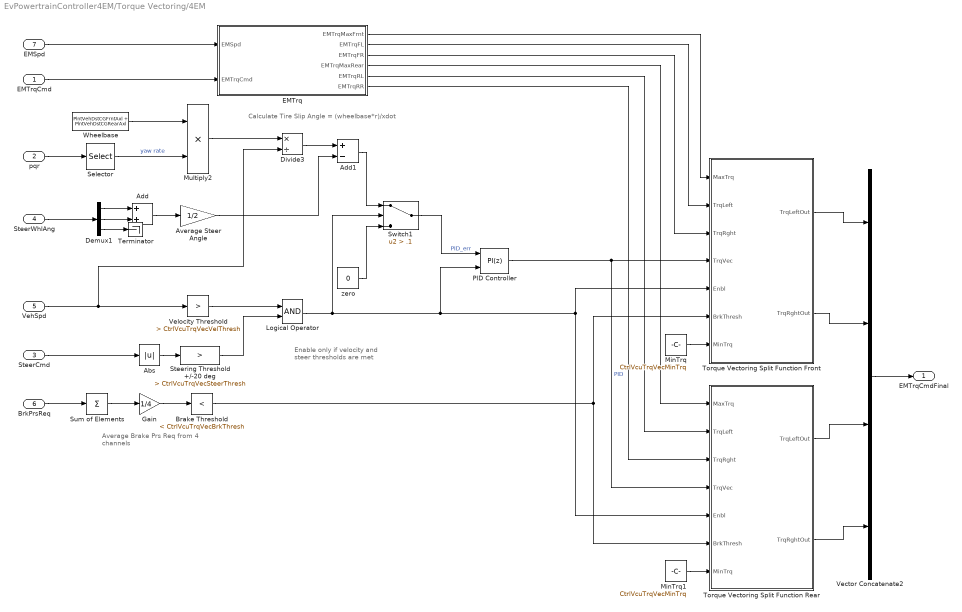
== system EvPowertrainController4EM/Torque Vectoring/4EM ==
  note: Average Brake Prs Req
      | from 4 channels
  note: Enable only if velocity and
      | steer thresholds are met
  note: Calculate Tire Slip Angle = (wheelbase*r)/xdot
  EMTrqCmd : Inport
  pqr : Inport  Port=2
  SteerCmd : Inport  Port=3
  SteerWhlAng : Inport  Port=4
  VehSpd : Inport  Port=5
  BrkPrsReq : Inport  Port=6
  EMSpd : Inport  Port=7
  Abs : Abs  SaturateOnIntegerOverflow=off
  Add : Sum
  Add1 : Sum  Inputs=+-
  Average Steer Angle : Gain  Gain=1/2
  Brake Threshold : simulink/Logic and Bit Operations/Compare To Constant  relop=<  const=CtrlVcuTrqVecBrkThresh  OutDataTypeStr=boolean
  Demux1 : Demux  Outputs=[1 1 2]
  Divide3 : Product  Inputs=*/
  EMTrq : Subsystem
  Gain : Gain  Gain=1/4
  Logical Operator : Logic  AllPortsSameDT=off  OutDataTypeStr=boolean
  MinTrq : Constant  Value=CtrlVcuTrqVecMinTrq  SampleTime=-1
  MinTrq1 : Constant  Value=CtrlVcuTrqVecMinTrq  SampleTime=-1
  Multiply2 : Product
  PID Controller : slpidlib/PID Controller  Controller=PI  Form=Parallel  TimeDomain=Discrete-time  UseExternalTs=off  SampleTime=-1  IntegratorMethod=Forward Euler  FilterMethod=Forward Euler  ControllerParametersSource=internal  P=CtrlVcuTrqVecPGain  I=CtrlVcuTrqVecPGain  UseKiTs=off  D=0  N=1  UseFilter=on  TunerSelectOption=Transfer Function Based (PID Tuner App)  ZeroCross=off  InitialConditionSource=internal  InitialConditionForIntegrator=0  InitialConditionForFilter=0  DifferentiatorICPrevScaledInput=0  ExternalReset=either  TrackingMode=off  Kt=1  LimitOutput=off  SatLimitsSource=internal  UpperSaturationLimit=inf  LowerSaturationLimit=-inf  LinearizeAsGain=on  AntiWindupMode=none  Kb=1  LimitIntegrator=off  UpperIntegratorSaturationLimit=inf  LowerIntegratorSaturationLimit=-inf  POutMin=[]  POutMax=[]  IOutMin=[]  IOutMax=[]  DOutMin=[]  DOutMax=[]  NOutMin=[]  NOutMax=[]  SumOutMin=[]  SumOutMax=[]  SaturationOutMin=[]  SaturationOutMax=[]  PParamMin=[]  PParamMax=[]  IParamMin=[]  IParamMax=[]  DParamMin=[]  DParamMax=[]  NParamMin=[]  NParamMax=[]  KbParamMin=[]  KbParamMax=[]  KtParamMin=[]  KtParamMax=[]  KbOutMin=[]  KbOutMax=[]  KtOutMin=[]  KtOutMax=[]  IntegratorOutMin=[]  IntegratorOutMax=[]  FilterOutMin=[]  FilterOutMax=[]  SumI1OutMin=[]  SumI1OutMax=[]  SumI2OutMin=[]  SumI2OutMax=[]  SumI3OutMin=[]  SumI3OutMax=[]  SumI4OutMin=[]  SumI4OutMax=[]  SumDOutMin=[]  SumDOutMax=[]  DifferentiatorOutMin=[]  DifferentiatorOutMax=[]  FilterDiffOutCoefMin=[]  FilterDiffOutCoefMax=[]  ReciprocalOutMin=[]  ReciprocalOutMax=[]  SumDenOutMin=[]  SumDenOutMax=[]  SumNumOutMin=[]  SumNumOutMax=[]  DivideOutMin=[]  DivideOutMax=[]  UdiffTsProdOutMin=[]  UdiffTsProdOutMax=[]  NTsProdOutMin=[]  NTsProdOutMax=[]  UintegralTsProdOutMin=[]  UintegralTsProdOutMax=[]  UngainTsProdOutMin=[]  UngainTsProdOutMax=[]  ClampingZeroOutDataTypeStr=Inherit: Inherit via back propagation  ClampingZeroOutMin=[]  ClampingZeroOutMax=[]  FilterDenConstantOutDataTypeStr=Inherit: Inherit via back propagation  FilterDenConstantOutMin=[]  FilterDenConstantOutMax=[]  PCopyOutDataTypeStr=Inherit: Inherit via back propagation  PCopyOutMin=[]  PCopyOutMax=[]  NCopyOutDataTypeStr=Inherit: Inherit via back propagation  NCopyOutMin=[]  NCopyOutMax=[]  IntegratorContinuousStateAttributes=''  IntegratorStateMustResolveToSignalObject=off  IntegratorRTWStateStorageClass=Auto  FilterContinuousStateAttributes=''  FilterStateMustResolveToSignalObject=off  FilterRTWStateStorageClass=Auto  ParallelPVariant=InternalParameters  IdealPVariant=Disabled  IVariant=InternalParameters  DVariant=Disabled  IntegratorVariant=Discrete  SatVariant=Disabled  AWVariant=Passthrough  PCopyVariant=Disabled  TRVariant=Disabled  FdbkBlocksVariant=Forward  IdealPFdbkVariant=Disabled  SatFdbkVariant=Disabled  DerivativeFilterVariant=Disabled  NVariant=Disabled  NCopyVariant=Disabled_SignalSpec  FilterICVariant=Disabled  IntegratorICVariant=InternalICs  ExternalResetVariant=ExternalReset  TRSumVariant=Passthrough  SumFdbkVariant=Disabled  SumVariant=Sum_PI  TsampFilterVariant=InternalTs  TsampNgainVariant=Passthrough  TsampIntegralVariant=Disabled_SignalSpec  ExternalSaturationOutDataTypeStr=Inherit: Same as second input
  Selector : Selector  InputPortWidth=3  IndexOptions=Index vector (dialog)  Indices=[3]  OutputSizes=1
  Steering Threshold +/-20 deg : simulink/Logic and Bit Operations/Compare To Constant  relop=>  const=CtrlVcuTrqVecSteerThresh  OutDataTypeStr=boolean
  Sum of Elements : Sum  Inputs=+
  Switch1 : Switch  Criteria=u2 > Threshold  Threshold=.1  SaturateOnIntegerOverflow=off  InputSameDT=off
  Terminator : Terminator
  Torque Vectoring Split Function Front : MATLAB Function  TreatAsAtomicUnit=on
  Torque Vectoring Split Function Rear : MATLAB Function  TreatAsAtomicUnit=on
  Vector Concatenate2 : Concatenate  NumInputs=4
  Velocity Threshold : simulink/Logic and Bit Operations/Compare To Constant  relop=>  const=CtrlVcuTrqVecVelThresh  OutDataTypeStr=boolean
  Wheelbase : Constant  Value=PlntVehDstCGFrntAxl + PlntVehDstCGRearAxl  SampleTime=-1
  zero : Constant  Value=0  SampleTime=-1
  EMTrqCmdFinal : Outport  VectorParamsAs1DForOutWhenUnconnected=off
  wires:
  EMTrqCmd/1 -> EMTrq/2(EMTrqCmd)
  Vector Concatenate2/1 -> EMTrqCmdFinal/1
  MinTrq/1 -> Torque Vectoring Split Function Front/7(MinTrq)
  Wheelbase/1 -> Multiply2/1
  Demux1/3 -> Terminator/1
  BrkPrsReq/1 -> Sum of Elements/1
  Divide3/1 -> Add1/1
  Switch1/1 -> PID Controller/1  "PID_err"
  SteerCmd/1 -> Abs/1
  Demux1/2 -> Add/2
  VehSpd/1 -> Velocity Threshold/1, Divide3/2
  Multiply2/1 -> Divide3/1
  Average Steer Angle/1 -> Add1/2
  PID Controller/1 -> Torque Vectoring Split Function Rear/4(TrqVec), Torque Vectoring Split Function Front/4(TrqVec)  "PID"
  Brake Threshold/1 -> Torque Vectoring Split Function Rear/6(BrkThresh), Torque Vectoring Split Function Front/6(BrkThresh)
  Logical Operator/1 -> PID Controller/2, Torque Vectoring Split Function Rear/5(Enbl), Torque Vectoring Split Function Front/5(Enbl), Switch1/2
  Torque Vectoring Split Function Front/2(TrqRghtOut) -> Vector Concatenate2/2
  Add/1 -> Average Steer Angle/1
  Steering Threshold +/-20 deg/1 -> Logical Operator/2
  Torque Vectoring Split Function Front/1(TrqLeftOut) -> Vector Concatenate2/1
  Abs/1 -> Steering Threshold +/-20 deg/1
  Velocity Threshold/1 -> Logical Operator/1
  Demux1/1 -> Add/1
  zero/1 -> Switch1/3
  pqr/1 -> Selector/1
  SteerWhlAng/1 -> Demux1/1
  Add1/1 -> Switch1/1
  EMSpd/1 -> EMTrq/1(EMSpd)
  EMTrq/1(EMTrqMaxFrnt) -> Torque Vectoring Split Function Front/1(MaxTrq)
  EMTrq/2(EMTrqFL) -> Torque Vectoring Split Function Front/2(TrqLeft)
  EMTrq/3(EMTrqFR) -> Torque Vectoring Split Function Front/3(TrqRght)
  Sum of Elements/1 -> Gain/1
  Gain/1 -> Brake Threshold/1
  Selector/1 -> Multiply2/2  "yaw rate"
  MinTrq1/1 -> Torque Vectoring Split Function Rear/7(MinTrq)
  EMTrq/4(EMTrqMaxRear) -> Torque Vectoring Split Function Rear/1(MaxTrq)
  EMTrq/5(EMTrqRL) -> Torque Vectoring Split Function Rear/2(TrqLeft)
  EMTrq/6(EMTrqRR) -> Torque Vectoring Split Function Rear/3(TrqRght)
  Torque Vectoring Split Function Rear/1(TrqLeftOut) -> Vector Concatenate2/3
  Torque Vectoring Split Function Rear/2(TrqRghtOut) -> Vector Concatenate2/4

== system EvPowertrainController4EM/Torque Vectoring/No Torque Vectoring ==
  EMTrqCmd : Inport
  EMTrqCmdFinal : Outport  VectorParamsAs1DForOutWhenUnconnected=off
  wires:
  EMTrqCmd/1 -> EMTrqCmdFinal/1

== system EvPowertrainController4EM/Accel Pedal to Traction Wheel Torque Request/EM2WhlTrq/2EM ==
  note: Reflect EMTrq to WhlTrq
      | due to possible gearing
      | differences
  note: Use VehSpd instead of EMSpd or
      | WhlSpd in case wheel or EM are
      | undergoing slipping / have oscillations.
  Gear : Inport
  VehSpd : Inport  Port=2
  Add : Sum
  EMTrq2WhlTrqFrnt : Subsystem  Variant=on  VariantControlMode=label  VariantControl=1  LabelModeActiveChoice=3
  EMTrq2WhlTrqRear : Subsystem  Variant=on  VariantControlMode=label  VariantControl=1  LabelModeActiveChoice=3
  Maximum Torque Front Axle : Subsystem
  Maximum Torque Rear Axle : Subsystem
  VehSpd2EMSpd : Subsystem  Variant=on  VariantControlMode=label  VariantControl=1  LabelModeActiveChoice=3
  WhlTrqCmd : Outport
  wires:
  Maximum Torque Front Axle/1(EMTrq) -> EMTrq2WhlTrqFrnt/2(EMTrqCmd)
  VehSpd2EMSpd/1(EMSpdFrntAxl) -> EMTrq2WhlTrqFrnt/3(EMSpd), Maximum Torque Front Axle/1(EMSpd)
  Maximum Torque Rear Axle/1(EMTrq) -> EMTrq2WhlTrqRear/2(EMTrqCmd)
  Gear/1 -> VehSpd2EMSpd/1(Gear), EMTrq2WhlTrqFrnt/1(Gear), EMTrq2WhlTrqRear/1(Gear)
  EMTrq2WhlTrqFrnt/1(WhlMotTrq) -> Add/1
  VehSpd/1 -> VehSpd2EMSpd/2(VehSpd)
  Add/1 -> WhlTrqCmd/1
  EMTrq2WhlTrqRear/1(WhlMotTrq) -> Add/2
  VehSpd2EMSpd/2(EMSpdRearAxl) -> EMTrq2WhlTrqRear/3(EMSpd), Maximum Torque Rear Axle/1(EMSpd)

== system EvPowertrainController4EM/Accel Pedal to Traction Wheel Torque Request/EM2WhlTrq/3EM Dual Front ==
  note: Use VehSpd instead of EMSpd or
      | WhlSpd in case wheel or EM are
      | undergoing slipping / have oscillations.
  note: Reflect EMTrq to WhlTrq
      | due to possible gearing
      | differences
  Gear : Inport
  VehSpd : Inport  Port=2
  Add : Sum
  EMTrq2WhlTrqFrnt : Subsystem  Variant=on  VariantControlMode=label  VariantControl=1  LabelModeActiveChoice=3
  EMTrq2WhlTrqRear : Subsystem  Variant=on  VariantControlMode=label  VariantControl=1  LabelModeActiveChoice=3
  Maximum Torque Front Axle : Subsystem
  Maximum Torque Rear Axle : Subsystem
  VehSpd2EMSpd : Subsystem  Variant=on  VariantControlMode=label  VariantControl=1  LabelModeActiveChoice=3
  WhlTrqCmd : Outport
  wires:
  VehSpd2EMSpd/2(EMSpdRearAxl) -> Maximum Torque Rear Axle/1(EMSpd), EMTrq2WhlTrqRear/3(EMSpd)
  EMTrq2WhlTrqRear/1(WhlMotTrq) -> Add/2
  Add/1 -> WhlTrqCmd/1
  VehSpd/1 -> VehSpd2EMSpd/2(VehSpd)
  EMTrq2WhlTrqFrnt/1(WhlMotTrq) -> Add/1
  Gear/1 -> EMTrq2WhlTrqRear/1(Gear), EMTrq2WhlTrqFrnt/1(Gear), VehSpd2EMSpd/1(Gear)
  Maximum Torque Rear Axle/1(EMTrq) -> EMTrq2WhlTrqRear/2(EMTrqCmd)
  VehSpd2EMSpd/1(EMSpdFrntAxl) -> Maximum Torque Front Axle/1(EMSpd), EMTrq2WhlTrqFrnt/3(EMSpd)
  Maximum Torque Front Axle/1(EMTrq) -> EMTrq2WhlTrqFrnt/2(EMTrqCmd)

== system EvPowertrainController4EM/Accel Pedal to Traction Wheel Torque Request/EM2WhlTrq/3EM Dual Rear ==
  note: Reflect EMTrq to WhlTrq
      | due to possible gearing
      | differences
  note: Use VehSpd instead of EMSpd or
      | WhlSpd in case wheel or EM are
      | undergoing slipping / have oscillations.
  Gear : Inport
  VehSpd : Inport  Port=2
  Add : Sum
  EMTrq2WhlTrqFrnt : Subsystem  Variant=on  VariantControlMode=label  VariantControl=1  LabelModeActiveChoice=3
  EMTrq2WhlTrqRear : Subsystem  Variant=on  VariantControlMode=label  VariantControl=1  LabelModeActiveChoice=3
  Maximum Torque Front Axle : Subsystem
  Maximum Torque Rear Axle : Subsystem
  VehSpd2EMSpd : Subsystem  Variant=on  VariantControlMode=label  VariantControl=1  LabelModeActiveChoice=3
  WhlTrqCmd : Outport
  wires:
  Maximum Torque Front Axle/1(EMTrq) -> EMTrq2WhlTrqFrnt/2(EMTrqCmd)
  VehSpd2EMSpd/1(EMSpdFrntAxl) -> EMTrq2WhlTrqFrnt/3(EMSpd), Maximum Torque Front Axle/1(EMSpd)
  Maximum Torque Rear Axle/1(EMTrq) -> EMTrq2WhlTrqRear/2(EMTrqCmd)
  Gear/1 -> VehSpd2EMSpd/1(Gear), EMTrq2WhlTrqFrnt/1(Gear), EMTrq2WhlTrqRear/1(Gear)
  EMTrq2WhlTrqFrnt/1(WhlMotTrq) -> Add/1
  VehSpd/1 -> VehSpd2EMSpd/2(VehSpd)
  Add/1 -> WhlTrqCmd/1
  EMTrq2WhlTrqRear/1(WhlMotTrq) -> Add/2
  VehSpd2EMSpd/2(EMSpdRearAxl) -> EMTrq2WhlTrqRear/3(EMSpd), Maximum Torque Rear Axle/1(EMSpd)

== system EvPowertrainController4EM/Accel Pedal to Traction Wheel Torque Request/EM2WhlTrq/4EM ==
  note: Use VehSpd instead of EMSpd or
      | WhlSpd in case wheel or EM are
      | undergoing slipping / have oscillations.
  note: Reflect EMTrq to WhlTrq
      | due to possible gearing
      | differences
  Gear : Inport
  VehSpd : Inport  Port=2
  Add : Sum
  EMTrq2WhlTrqFrnt : Subsystem  Variant=on  VariantControlMode=label  VariantControl=1  LabelModeActiveChoice=3
  EMTrq2WhlTrqRear : Subsystem  Variant=on  VariantControlMode=label  VariantControl=1  LabelModeActiveChoice=3
  Maximum Torque Front Axle : Subsystem
  Maximum Torque Rear Axle : Subsystem
  VehSpd2EMSpd : Subsystem  Variant=on  VariantControlMode=label  VariantControl=1  LabelModeActiveChoice=3
  WhlTrqCmd : Outport
  wires:
  VehSpd2EMSpd/2(EMSpdRearAxl) -> Maximum Torque Rear Axle/1(EMSpd), EMTrq2WhlTrqRear/3(EMSpd)
  EMTrq2WhlTrqRear/1(WhlMotTrq) -> Add/2
  Add/1 -> WhlTrqCmd/1
  VehSpd/1 -> VehSpd2EMSpd/2(VehSpd)
  EMTrq2WhlTrqFrnt/1(WhlMotTrq) -> Add/1
  Gear/1 -> EMTrq2WhlTrqRear/1(Gear), EMTrq2WhlTrqFrnt/1(Gear), VehSpd2EMSpd/1(Gear)
  Maximum Torque Rear Axle/1(EMTrq) -> EMTrq2WhlTrqRear/2(EMTrqCmd)
  VehSpd2EMSpd/1(EMSpdFrntAxl) -> Maximum Torque Front Axle/1(EMSpd), EMTrq2WhlTrqFrnt/3(EMSpd)
  Maximum Torque Front Axle/1(EMTrq) -> EMTrq2WhlTrqFrnt/2(EMTrqCmd)

== system EvPowertrainController4EM/Energy Management/Calculate Average EMSpd and Wheel Torque Curves for Front and Rear Axles/2EM ==
  note: Reflect EMTrq to WhlTrq
      | due to possible gearing
      | differences
  EMSpd : Inport
  Gear : Inport  Port=2
  EMTrq2WhlTrqFrnt : Subsystem  Variant=on  VariantControlMode=label  VariantControl=1  LabelModeActiveChoice=3
  EMTrq2WhlTrqRear : Subsystem  Variant=on  VariantControlMode=label  VariantControl=1  LabelModeActiveChoice=3
  Maximum Torque Front Axle : Subsystem
  Maximum Torque Rear Axle : Subsystem
  Selector : Selector  InputPortWidth=2  IndexOptions=Index vector (dialog)  Indices=[1]  OutputSizes=1
  Selector1 : Selector  InputPortWidth=2  IndexOptions=Index vector (dialog)  Indices=[2]  OutputSizes=1
  Vector Concatenate : Concatenate
  Vector Concatenate1 : Concatenate
  EMAvgSpdVec : Outport
  WhlTrqMaxVec : Outport  Port=2
  wires:
  EMSpd/1 -> Selector/1, Selector1/1
  Selector1/1 -> Vector Concatenate1/2, EMTrq2WhlTrqRear/3(EMSpd), Maximum Torque Rear Axle/1(EMSpd)
  EMTrq2WhlTrqRear/1(WhlMotTrq) -> Vector Concatenate/2
  Gear/1 -> EMTrq2WhlTrqFrnt/1(Gear), EMTrq2WhlTrqRear/1(Gear)
  Selector/1 -> Vector Concatenate1/1, EMTrq2WhlTrqFrnt/3(EMSpd), Maximum Torque Front Axle/1(EMSpd)
  EMTrq2WhlTrqFrnt/1(WhlMotTrq) -> Vector Concatenate/1
  Maximum Torque Rear Axle/1(EMTrq) -> EMTrq2WhlTrqRear/2(EMTrqCmd)
  Maximum Torque Front Axle/1(EMTrq) -> EMTrq2WhlTrqFrnt/2(EMTrqCmd)
  Vector Concatenate/1 -> WhlTrqMaxVec/1
  Vector Concatenate1/1 -> EMAvgSpdVec/1

== system EvPowertrainController4EM/Energy Management/Calculate Average EMSpd and Wheel Torque Curves for Front and Rear Axles/3EM Dual Front ==
  note: Calculate average speed
      | of EMs on axle
  note: Reflect EMTrq to WhlTrq
      | due to possible gearing
      | differences
  EMSpd : Inport
  Gear : Inport  Port=2
  EMTrq2WhlTrqFrnt : Subsystem  Variant=on  VariantControlMode=label  VariantControl=1  LabelModeActiveChoice=3
  EMTrq2WhlTrqRear : Subsystem  Variant=on  VariantControlMode=label  VariantControl=1  LabelModeActiveChoice=3
  Gain : Gain  Gain=1/2
  Maximum Torque Front Axle : Subsystem
  Maximum Torque Rear Axle : Subsystem
  Selector : Selector  InputPortWidth=3  IndexOptions=Index vector (dialog)  Indices=[1 2]  OutputSizes=1
  Selector1 : Selector  InputPortWidth=3  IndexOptions=Index vector (dialog)  Indices=[3]  OutputSizes=1
  Sum of Elements : Sum  Inputs=+
  Vector Concatenate : Concatenate
  Vector Concatenate1 : Concatenate
  EMAvgSpdVec : Outport
  WhlTrqMaxVec : Outport  Port=2
  wires:
  Selector/1 -> Sum of Elements/1
  EMSpd/1 -> Selector1/1, Selector/1
  Sum of Elements/1 -> Gain/1
  Maximum Torque Rear Axle/1(EMTrq) -> EMTrq2WhlTrqRear/2(EMTrqCmd)
  Maximum Torque Front Axle/1(EMTrq) -> EMTrq2WhlTrqFrnt/2(EMTrqCmd)
  Gain/1 -> Vector Concatenate1/1, EMTrq2WhlTrqFrnt/3(EMSpd), Maximum Torque Front Axle/1(EMSpd)
  Gear/1 -> EMTrq2WhlTrqRear/1(Gear), EMTrq2WhlTrqFrnt/1(Gear)
  Selector1/1 -> Maximum Torque Rear Axle/1(EMSpd), EMTrq2WhlTrqRear/3(EMSpd), Vector Concatenate1/2
  EMTrq2WhlTrqRear/1(WhlMotTrq) -> Vector Concatenate/2
  EMTrq2WhlTrqFrnt/1(WhlMotTrq) -> Vector Concatenate/1
  Vector Concatenate/1 -> WhlTrqMaxVec/1
  Vector Concatenate1/1 -> EMAvgSpdVec/1

== system EvPowertrainController4EM/Energy Management/Calculate Average EMSpd and Wheel Torque Curves for Front and Rear Axles/3EM Dual Rear ==
  note: Calculate average speed
      | of EMs on axle
  note: Reflect EMTrq to WhlTrq
      | due to possible gearing
      | differences
  EMSpd : Inport
  Gear : Inport  Port=2
  EMTrq2WhlTrqFrnt : Subsystem  Variant=on  VariantControlMode=label  VariantControl=1  LabelModeActiveChoice=3
  EMTrq2WhlTrqRear : Subsystem  Variant=on  VariantControlMode=label  VariantControl=1  LabelModeActiveChoice=3
  Gain : Gain  Gain=1/2
  Maximum Torque Front Axle : Subsystem
  Maximum Torque Rear Axle : Subsystem
  Selector : Selector  InputPortWidth=3  IndexOptions=Index vector (dialog)  Indices=[2 3]  OutputSizes=1
  Selector1 : Selector  InputPortWidth=3  IndexOptions=Index vector (dialog)  Indices=[1]  OutputSizes=1
  Sum of Elements : Sum  Inputs=+
  Vector Concatenate : Concatenate
  Vector Concatenate1 : Concatenate
  EMAvgSpdVec : Outport
  WhlTrqMaxVec : Outport  Port=2
  wires:
  Sum of Elements/1 -> Gain/1
  EMSpd/1 -> Selector1/1, Selector/1
  Selector/1 -> Sum of Elements/1
  EMTrq2WhlTrqRear/1(WhlMotTrq) -> Vector Concatenate/2
  Gain/1 -> Vector Concatenate1/2, EMTrq2WhlTrqRear/3(EMSpd), Maximum Torque Rear Axle/1(EMSpd)
  Maximum Torque Rear Axle/1(EMTrq) -> EMTrq2WhlTrqRear/2(EMTrqCmd)
  Maximum Torque Front Axle/1(EMTrq) -> EMTrq2WhlTrqFrnt/2(EMTrqCmd)
  Selector1/1 -> Vector Concatenate1/1, EMTrq2WhlTrqFrnt/3(EMSpd), Maximum Torque Front Axle/1(EMSpd)
  Gear/1 -> EMTrq2WhlTrqFrnt/1(Gear), EMTrq2WhlTrqRear/1(Gear)
  EMTrq2WhlTrqFrnt/1(WhlMotTrq) -> Vector Concatenate/1
  Vector Concatenate/1 -> WhlTrqMaxVec/1
  Vector Concatenate1/1 -> EMAvgSpdVec/1

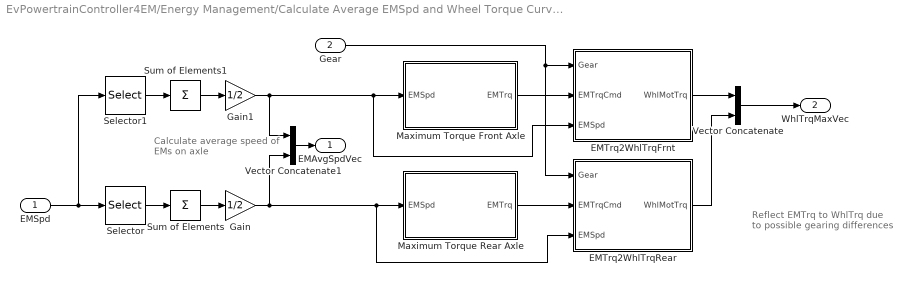
== system EvPowertrainController4EM/Energy Management/Calculate Average EMSpd and Wheel Torque Curves for Front and Rear Axles/4EM ==
  note: Calculate average speed
      | of EMs on axle
  note: Reflect EMTrq to WhlTrq
      | due to possible gearing
      | differences
  EMSpd : Inport
  Gear : Inport  Port=2
  EMTrq2WhlTrqFrnt : Subsystem  Variant=on  VariantControlMode=label  VariantControl=1  LabelModeActiveChoice=3
  EMTrq2WhlTrqRear : Subsystem  Variant=on  VariantControlMode=label  VariantControl=1  LabelModeActiveChoice=3
  Gain : Gain  Gain=1/2
  Gain1 : Gain  Gain=1/2
  Maximum Torque Front Axle : Subsystem
  Maximum Torque Rear Axle : Subsystem
  Selector : Selector  InputPortWidth=4  IndexOptions=Index vector (dialog)  Indices=[3 4]  OutputSizes=1
  Selector1 : Selector  InputPortWidth=4  IndexOptions=Index vector (dialog)  Indices=[1 2]  OutputSizes=1
  Sum of Elements : Sum  Inputs=+
  Sum of Elements1 : Sum  Inputs=+
  Vector Concatenate : Concatenate
  Vector Concatenate1 : Concatenate
  EMAvgSpdVec : Outport
  WhlTrqMaxVec : Outport  Port=2
  wires:
  Selector/1 -> Sum of Elements/1
  Selector1/1 -> Sum of Elements1/1
  EMSpd/1 -> Selector/1, Selector1/1
  Sum of Elements/1 -> Gain/1
  Sum of Elements1/1 -> Gain1/1
  EMTrq2WhlTrqRear/1(WhlMotTrq) -> Vector Concatenate/2
  Maximum Torque Front Axle/1(EMTrq) -> EMTrq2WhlTrqFrnt/2(EMTrqCmd)
  Maximum Torque Rear Axle/1(EMTrq) -> EMTrq2WhlTrqRear/2(EMTrqCmd)
  Gain1/1 -> Vector Concatenate1/1, EMTrq2WhlTrqFrnt/3(EMSpd), Maximum Torque Front Axle/1(EMSpd)
  EMTrq2WhlTrqFrnt/1(WhlMotTrq) -> Vector Concatenate/1
  Gear/1 -> EMTrq2WhlTrqRear/1(Gear), EMTrq2WhlTrqFrnt/1(Gear)
  Gain/1 -> Vector Concatenate1/2, Maximum Torque Rear Axle/1(EMSpd), EMTrq2WhlTrqRear/3(EMSpd)
  Vector Concatenate/1 -> WhlTrqMaxVec/1
  Vector Concatenate1/1 -> EMAvgSpdVec/1

== system EvPowertrainController4EM/Energy Management/Control Domain /Rear Axle EM Torque Vector ==
  EMAvgSpdVec : Inport
  2EM or 3EM Dual Front : Subsystem  VariantControl=2EM or 3EM Dual Front
  3EM Dual Rear or 4EM : Subsystem  VariantControl=3EM Dual Rear or 4EM
  WhlEMRearVecPos : Outport
  WhlEMRearVecNeg : Outport  Port=2
